simulink model "pitch_rate_feedback"  (Simulink 7.7)
settings: Solver=ode45  StartTime=0.0  StopTime=30.0  RelTol=1e-3
PreLoadFcn:
  | load 'linearized_num.mat'
  | load 'linearized_den.mat'
values from neighbouring files (symbols this model uses):
  den = [1 4.58030539277 13.8482324239 0.423666561847 1.0363236974]    [linearized_den.mat]
  num = [0 0 0 0 -0.013605000831 -0.824066014405 -0.327489589552 0 -0.0937383605768 -57.5305207591 -0.761123497998 -0.327489589552 ... (20 elements, 4x5)]    [linearized_num.mat]
settings Model: Creator=Home  LastModifiedBy=ggramajo

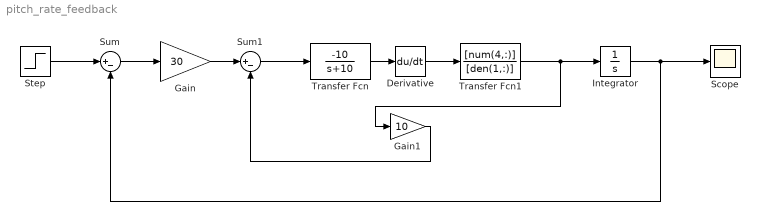
== system pitch_rate_feedback ==
  Derivative : Derivative
  Gain : Gain  Gain=30
  Gain1 : Gain  Gain=10
  Integrator : Integrator
  Scope : Scope
  Step : Step  After=5*pi/180  SampleTime=0
  Sum : Sum  Inputs=|+-
  Sum1 : Sum  Inputs=|+-
  Transfer Fcn : TransferFcn  Numerator=[-10]  Denominator=[1 10]
  Transfer Fcn1 : TransferFcn  Numerator=[num(4,:)]  Denominator=[den(1,:)]
  wires:
  Step/1 -> Sum/1
  Transfer Fcn/1 -> Derivative/1
  Transfer Fcn1/1 -> Integrator/1, Gain1/1
  Integrator/1 -> Scope/1, Sum/2
  Derivative/1 -> Transfer Fcn1/1
  Sum/1 -> Gain/1
  Gain/1 -> Sum1/1
  Sum1/1 -> Transfer Fcn/1
  Gain1/1 -> Sum1/2
